simulink model "gridMapModel_TCPIP"  (R2014a)
settings: Solver=ode45  StartTime=0.0  StopTime=Inf  RelTol=1e-3
InitFcn:
  | close all;
  | 
  | lid = LIDAR();
  | rob = DifferentialRobot();
  | rob.dt = 0.02;
  | rob.attachLidar(lid, [0.6,0,0]);
  | 
  | subplot(1, 2, 1);
  | gm = GridMap([60 40], 0.1);
  | ghMap = imshow(gm.map);
  | 
  | 
  | ghPlot =subplot(1, 2, 2);
  | hold on;
  | axis equal;
  | hold on;
  | whitebg([0 0 0]);
  | grid on;
  | pl = Plotter(ghPlot);
libraries: iWalkerLib x1
settings Model: Creator=Brian  LastModifiedBy=Brian

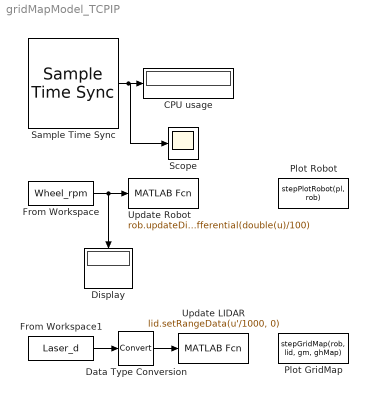
== system gridMapModel_TCPIP ==
  CPU usage : Display
  Data Type Conversion : DataTypeConversion
  Display : Display
  From Workspace : FromWorkspace  VariableName=Wheel_rpm  SampleTime=0.02  Interpolate=off  OutputAfterFinalValue=Setting to zero
  From Workspace1 : FromWorkspace  VariableName=Laser_d  SampleTime=0.4  Interpolate=off  OutputAfterFinalValue=Setting to zero
  Plot GridMap : MATLABFcn  MATLABFcn=stepGridMap(rob, lid, gm, ghMap)  OutputDimensions=0  SampleTime=1
  Plot Robot : MATLABFcn  MATLABFcn=stepPlotRobot(pl, rob)  OutputDimensions=0  SampleTime=1/30
  Sample Time Sync : iWalkerLib/Sample Time Sync  Priority=8
  Scope : Scope
      settings: YMin=0  YMax=22500
  Update LIDAR : MATLABFcn  MATLABFcn=lid.setRangeData(u'/1000, 0)  OutputDimensions=0
  Update Robot : MATLABFcn  MATLABFcn=rob.updateDifferential(double(u)/100)  OutputDimensions=0
  wires:
  From Workspace/1 -> Update Robot/1, Display/1
  From Workspace1/1 -> Data Type Conversion/1
  Sample Time Sync/1 -> Scope/1, CPU usage/1
  Data Type Conversion/1 -> Update LIDAR/1
